simulink model "MeasModelCompare_exh"  (R2014b)
settings: Solver=ode45  StartTime=0.0  StopTime=10.0  RelTol=1e-3
values from neighbouring files (symbols this model uses):
  AirStep =     [AirStep.mat]
  tau_th = 0.032    [Init_Project1.m]
settings Model: Creator=danfa688  LastModifiedBy=danfa688

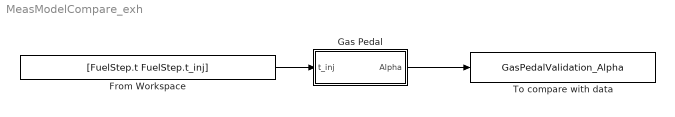
== system MeasModelCompare_exh ==
  From Workspace : FromWorkspace  VariableName=[FuelStep.t FuelStep.t_inj]  SampleTime=0
  Gas Pedal : Subsystem
  To compare with data : ToWorkspace  VariableName=GasPedalValidation_Alpha  SaveFormat=Structure With Time  SampleTime=-1
  wires:
  Gas Pedal/1(Alpha) -> To compare with data/1
  From Workspace/1 -> Gas Pedal/1(t_inj)

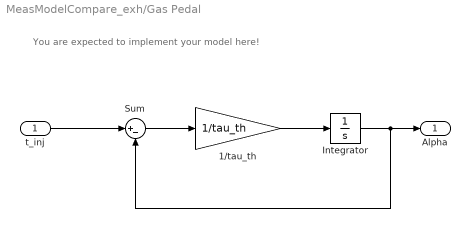
== system MeasModelCompare_exh/Gas Pedal ==
  note: You are expected to implement your model here!
  t_inj : Inport
  1/tau_th : Gain  Gain=1/tau_th  SaturateOnIntegerOverflow=on  OutDataTypeStr=Inherit: Same as input  ParamDataTypeStr=Inherit: Same as input
  Integrator : Integrator  InitialCondition=AirStep.alpha_ref(1)
  Sum : Sum  Inputs=|+-  SaturateOnIntegerOverflow=on
  Alpha : Outport
  wires:
  t_inj/1 -> Sum/1
  Sum/1 -> 1/tau_th/1
  Integrator/1 -> Alpha/1, Sum/2
  1/tau_th/1 -> Integrator/1
